simulink model "v05DCMotorHarmonicDriveTemperatureDependent"  (R2016b)
settings: Solver=VariableStepAuto  StartTime=0.0  StopTime=0.1  RelTol=1e-3  AbsTol=1e-3  EnableMultiTasking=on
values from neighbouring files (symbols this model uses):
  J_rotor = 1    [v05DCMotorHarmonicDriveTemperatureDependentScript.m]
  K_t = 0.044415    [v05DCMotorHarmonicDriveTemperatureDependentScript.m]
  V_in = 20    [v05DCMotorHarmonicDriveTemperatureDependentScript.m]
libraries: fl_lib x20, nesl_utility x10, elec_lib x1, sdl_lib x1, simulink x1
settings Model: Creator=Taeke  LastModifiedBy=Taeke
settings DataIOCC: LimitDataPoints=on
settings OptimizationCC: LifeSpan=inf
settings DebuggingCC: AllowSymbolicDim=off  SFUnexpectedBacktrackingDiag=warning  SFNoUnconditionalDefaultTransitionDiag=warning  SFExecutionAtInitializationDiag=none
settings GRTTargetCC: TargetLangStandard=C89/C90 (ANSI)  GeneratePreprocessorConditionals=Disable all
settings ConfigComp: CovMetricSettings=dw  CovHtmlReporting=on  CovSaveCumulativeToWorkspaceVar=on  CovSaveSingleToWorkspaceVar=on  CovExternalEMLEnable=off  CovSFcnEnable=off
settings SimscapeCC: SimscapeLogType=all  SimscapeLogDataHistory=10000

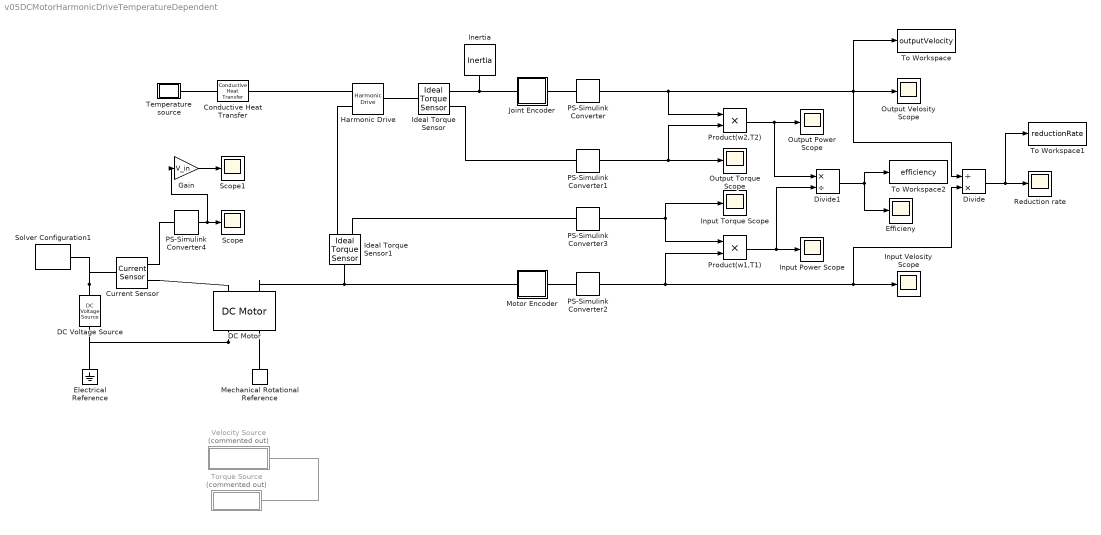
== system v05DCMotorHarmonicDriveTemperatureDependent ==
  Conductive Heat Transfer : fl_lib/Thermal/Thermal Elements/Conductive Heat Transfer  area=1 m^2  thickness=0.1 m  th_cond=401 W/(m*K)  Q_specify=off  Q_priority=None  Q=0 J/s  T_specify=off  T_priority=None  T=0 K
  Current Sensor : fl_lib/Electrical/Electrical Sensors/Current Sensor
  DC Motor : elec_lib/Actuators & Drivers/Rotational Actuators/DC Motor  parameterization=1  Ra=R_armat Ohm  La=H_armat H  emf_or_torque=2  Kv=7.2e-5 V/rpm  Ki=K_t N*m/A  T_stall=2.4e-4 N*m  w_max=1.91e+4 rpm  w_rated=1.5e+4 rpm  P_rated=0.08 W  V_rated=1.5 V  J=J_rotor g*cm^2  lam_param=1  lam=0 N*m/(rad/s)  i_noload=0 A  V_i_noload=1.5 V  speed0=0 rpm  alpha=0.00393 1/K  Tmeas=25 degC  thermal_mass=100 J/K  initial_temperature=25 degC
  DC Voltage Source : fl_lib/Electrical/Electrical Sources/DC Voltage Source  v0=V_in V
  Divide : Product  Inputs=/*
  Divide1 : Product  Inputs=*/
  Efficieny : Scope
  Electrical Reference : fl_lib/Electrical/Electrical Elements/Electrical Reference
  Gain : Gain  Gain=V_in
  Harmonic Drive : sdl_lib/Gears/Harmonic Drive  n_ellipse=N_teeth_elip  n_circle=N_teeth_circ  friction_model=1  T_noload=0.01 N*m  T_nom=0.1 N*m  efficiency_nom=.75  efficiency=0.95  mu_visc=mu N*m/(rad/s)  w_thr=0.001 rad/s  pwr_thr=P_threshold W  temperature_TLU=T_efficiency K  load_TLU=[1.0, 5.0, 10.0] N*m  efficiency_TLU=etha_efficiency  efficiency_TLU2=[0.85, 0.8, 0.75; 0.95, 0.9, 0.85; 0.85, 0.8, 0.7]  thermal_mass=C_thermal J/K  T_init=T_initial K
  Ideal Torque Sensor : fl_lib/Mechanical/Mechanical Sensors/Ideal Torque Sensor
  Ideal Torque Sensor1 : fl_lib/Mechanical/Mechanical Sensors/Ideal Torque Sensor
  Inertia : fl_lib/Mechanical/Rotational Elements/Inertia  inertia=I_load kg*m^2  w_specify=on  w_priority=High  w=0 rad/s  t_specify=off  t_priority=None  t=0 N*m
  Input Power Scope : Scope
  Input Torque Scope : Scope
  Input Velosity Scope : Scope
  Joint Encoder : Subsystem
  Mechanical Rotational Reference : fl_lib/Mechanical/Rotational Elements/Mechanical Rotational Reference
  Motor Encoder : Subsystem
  Output Power Scope : Scope
  Output Torque Scope : Scope
  Output Velosity Scope : Scope
  PS-Simulink Converter : nesl_utility/PS-Simulink Converter  PhysicalDomain=network_engine_domain  SubClassName=ps_output  LeftPortType=input  RightPortType=output  PseudoPeriodic=off  Frequencies=[]  Unit=rad/s  AffineConversion=off
  PS-Simulink Converter1 : nesl_utility/PS-Simulink Converter  PhysicalDomain=network_engine_domain  SubClassName=ps_output  LeftPortType=input  RightPortType=output  PseudoPeriodic=off  Frequencies=[]  Unit=N*m  AffineConversion=off
  PS-Simulink Converter2 : nesl_utility/PS-Simulink Converter  PhysicalDomain=network_engine_domain  SubClassName=ps_output  LeftPortType=input  RightPortType=output  PseudoPeriodic=off  Frequencies=[]  Unit=rad/s  AffineConversion=off
  PS-Simulink Converter3 : nesl_utility/PS-Simulink Converter  PhysicalDomain=network_engine_domain  SubClassName=ps_output  LeftPortType=input  RightPortType=output  PseudoPeriodic=off  Frequencies=[]  Unit=N*m  AffineConversion=off
  PS-Simulink Converter4 : nesl_utility/PS-Simulink Converter  PhysicalDomain=network_engine_domain  SubClassName=ps_output  LeftPortType=input  RightPortType=output  PseudoPeriodic=off  Frequencies=[]  Unit=A  AffineConversion=off
  Product(w1,T1) : Product
  Product(w2,T2) : Product
  Reduction rate : Scope
  Scope : Scope
  Scope1 : Scope
  Solver Configuration1 : nesl_utility/Solver Configuration  PhysicalDomain=network_engine_domain  SubClassName=solver  LeftPortType=input  RightPortType=generic  Accelerate=off  Tones=[]  Harmonics=[]  SimulateNoise=off  Profile=off  UseLocalSampling=off  EnableSwitchedLinearOptims=on  FrequencyDomain=off  UseCCode=off  RelTol=0.001  AbsTol=1e-06  MinStep=1e-09  ToWorkspace=off  RevertToSquareIcSolve=off  NumHomotopyIterations=100  PhasorMode=off  PhasorModeNumHarmonics=1  OverrideAbsTol=off  DoDC=off  ResidualTolerance=1e-09  UseLocalSolver=off  LocalSolverChoice=NE_BACKWARD_EULER_ADVANCER  LocalSolverSampleTime=0.001  DoFixedCost=off  MaxNonlinIter=3  MaxModeIter=2  LinearAlgebra=Sparse  DelaysMemoryBudget=1024  AutomaticFiltering=on  FilteringTimeConstant=0.001
  Temperature source : Subsystem  mask{Temperature=320}
      mask prompts: Temperature "Temperature [K]"
  To Workspace : ToWorkspace  VariableName=outputVelocity  SaveFormat=Timeseries  SampleTime=-1
  To Workspace1 : ToWorkspace  VariableName=reductionRate  SaveFormat=Timeseries  SampleTime=-1
  To Workspace2 : ToWorkspace  VariableName=efficiency  SaveFormat=Timeseries  SampleTime=-1
  Torque Source : Subsystem  Commented=on  mask(Rotation Velocity Source){inputTorque=2}
      mask prompts: inputTorque "Constant Torque [Nm]"
      mask help: A source which generate a constant rotational velocity.
      mask init:
      | initialVelocity = 0;
  Velocity Source : Subsystem  Commented=on  mask(Rotation Velocity Source){inputVelocity=1000}
      mask prompts: inputVelocity "Constant Velosity [rad/s]"
      mask help: A source which generate a constant rotational velocity.
      mask init:
      | initialVelocity = 0;
  wires:
  PS-Simulink Converter/1 -> Product(w2,T2)/1, Output Velosity Scope/1, To Workspace/1, Divide/1
  Divide/1 -> To Workspace1/1, Reduction rate/1
  PS-Simulink Converter2/1 -> Product(w1,T1)/2, Divide/2, Input Velosity Scope/1
  PS-Simulink Converter1/1 -> Product(w2,T2)/2, Output Torque Scope/1
  PS-Simulink Converter3/1 -> Input Torque Scope/1, Product(w1,T1)/1
  Product(w1,T1)/1 -> Divide1/2, Input Power Scope/1
  Product(w2,T2)/1 -> Divide1/1, Output Power Scope/1
  Divide1/1 -> To Workspace2/1, Efficieny/1
  PS-Simulink Converter4/1 -> Gain/1, Scope/1
  Gain/1 -> Scope1/1
  connections:
  Joint Encoder/LConn1 -- Ideal Torque Sensor/RConn1 -- Inertia/LConn1
  Joint Encoder/RConn1 -- PS-Simulink Converter/LConn1
  Motor Encoder/RConn1 -- PS-Simulink Converter2/LConn1
  Harmonic Drive/RConn1 -- Ideal Torque Sensor/LConn1
  Ideal Torque Sensor/RConn2 -- PS-Simulink Converter1/LConn1
  Ideal Torque Sensor1/RConn1 -- Harmonic Drive/LConn1
  Ideal Torque Sensor1/RConn2 -- PS-Simulink Converter3/LConn1
  Ideal Torque Sensor1/LConn1 -- DC Motor/LConn2 -- Motor Encoder/LConn1
  Conductive Heat Transfer/LConn1 -- Temperature source/RConn1
  Conductive Heat Transfer/RConn1 -- Harmonic Drive/LConn2
  DC Motor/RConn1 -- DC Voltage Source/RConn1 -- Electrical Reference/LConn1
  Mechanical Rotational Reference/LConn1 -- DC Motor/RConn2
  DC Voltage Source/LConn1 -- Solver Configuration1/RConn1 -- Current Sensor/LConn1
  Current Sensor/RConn2 -- DC Motor/LConn1
  Current Sensor/RConn1 -- PS-Simulink Converter4/LConn1
  Velocity Source/LConn1 -- Torque Source/LConn1

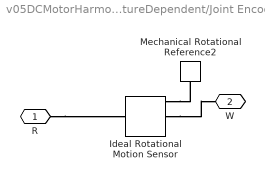
== system v05DCMotorHarmonicDriveTemperatureDependent/Joint Encoder ==
  Ideal Rotational Motion Sensor : fl_lib/Mechanical/Mechanical Sensors/Ideal Rotational Motion Sensor  offset=0 rad
  Mechanical Rotational Reference2 : fl_lib/Mechanical/Rotational Elements/Mechanical Rotational Reference
  R : PMIOPort  Port=1  Side=Left
  W : PMIOPort  Port=2  Side=Right
  connections:
  R/RConn1 -- Ideal Rotational Motion Sensor/LConn1
  Ideal Rotational Motion Sensor/RConn1 -- Mechanical Rotational Reference2/LConn1
  Ideal Rotational Motion Sensor/RConn2 -- W/RConn1

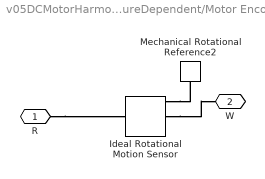
== system v05DCMotorHarmonicDriveTemperatureDependent/Motor Encoder ==
  Ideal Rotational Motion Sensor : fl_lib/Mechanical/Mechanical Sensors/Ideal Rotational Motion Sensor  offset=0 rad
  Mechanical Rotational Reference2 : fl_lib/Mechanical/Rotational Elements/Mechanical Rotational Reference
  R : PMIOPort  Port=1  Side=Left
  W : PMIOPort  Port=2  Side=Right
  connections:
  R/RConn1 -- Ideal Rotational Motion Sensor/LConn1
  Ideal Rotational Motion Sensor/RConn1 -- Mechanical Rotational Reference2/LConn1
  Ideal Rotational Motion Sensor/RConn2 -- W/RConn1

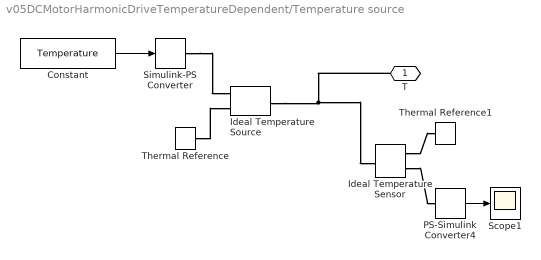
== system v05DCMotorHarmonicDriveTemperatureDependent/Temperature source ==
  Constant : Constant  Value=Temperature
  Ideal Temperature Sensor : fl_lib/Thermal/Thermal Sensors/Ideal Temperature Sensor
  Ideal Temperature Source : fl_lib/Thermal/Thermal Sources/Ideal Temperature Source
  PS-Simulink Converter4 : nesl_utility/PS-Simulink Converter  PhysicalDomain=network_engine_domain  SubClassName=ps_output  LeftPortType=input  RightPortType=output  PseudoPeriodic=off  Frequencies=[]  Unit=1  AffineConversion=off
  Scope1 : Scope
  Simulink-PS Converter : nesl_utility/Simulink-PS Converter  PhysicalDomain=network_engine_domain  SubClassName=ps_input  LeftPortType=input  RightPortType=output  PseudoPeriodic=off  Frequencies=[]  NoiseDistribution=none  NoiseParameters=[]  Unit=1  AffineConversion=off  InputFiltering=off  SimscapeFilterOrder=1  InputFilterTimeConstant=0.001  UdotUserProvided=1
  Thermal Reference : fl_lib/Thermal/Thermal Elements/Thermal Reference
  Thermal Reference1 : fl_lib/Thermal/Thermal Elements/Thermal Reference
  T : PMIOPort  Port=1  Side=Right
  wires:
  Constant/1 -> Simulink-PS Converter/1
  PS-Simulink Converter4/1 -> Scope1/1
  connections:
  Ideal Temperature Sensor/RConn1 -- Thermal Reference1/LConn1
  Simulink-PS Converter/RConn1 -- Ideal Temperature Source/RConn1
  Ideal Temperature Source/LConn1 -- T/RConn1 -- Ideal Temperature Sensor/LConn1
  Thermal Reference/LConn1 -- Ideal Temperature Source/RConn2
  Ideal Temperature Sensor/RConn2 -- PS-Simulink Converter4/LConn1

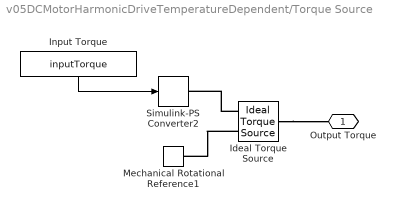
== system v05DCMotorHarmonicDriveTemperatureDependent/Torque Source ==
  Ideal Torque Source : fl_lib/Mechanical/Mechanical Sources/Ideal Torque Source
  Input Torque : Constant  Value=inputTorque
  Mechanical Rotational Reference1 : fl_lib/Mechanical/Rotational Elements/Mechanical Rotational Reference
  Simulink-PS Converter2 : nesl_utility/Simulink-PS Converter  PhysicalDomain=network_engine_domain  SubClassName=ps_input  LeftPortType=input  RightPortType=output  PseudoPeriodic=off  Frequencies=[]  NoiseDistribution=none  NoiseParameters=[]  Unit=1  AffineConversion=off  InputFiltering=off  SimscapeFilterOrder=1  InputFilterTimeConstant=0.001  UdotUserProvided=1
  Output Torque : PMIOPort  Port=1  Side=Left
  wires:
  Input Torque/1 -> Simulink-PS Converter2/1
  connections:
  Ideal Torque Source/RConn1 -- Simulink-PS Converter2/RConn1
  Ideal Torque Source/RConn2 -- Mechanical Rotational Reference1/LConn1
  Ideal Torque Source/LConn1 -- Output Torque/RConn1

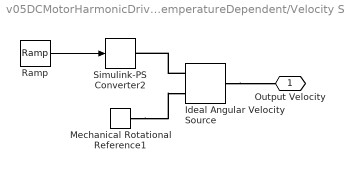
== system v05DCMotorHarmonicDriveTemperatureDependent/Velocity Source ==
  Ideal Angular Velocity Source : fl_lib/Mechanical/Mechanical Sources/Ideal Angular Velocity Source
  Mechanical Rotational Reference1 : fl_lib/Mechanical/Rotational Elements/Mechanical Rotational Reference
  Ramp : simulink/Sources/Ramp  slope=100  start=0  X0=0
  Simulink-PS Converter2 : nesl_utility/Simulink-PS Converter  PhysicalDomain=network_engine_domain  SubClassName=ps_input  LeftPortType=input  RightPortType=output  PseudoPeriodic=off  Frequencies=[]  NoiseDistribution=none  NoiseParameters=[]  Unit=1  AffineConversion=off  InputFiltering=on  SimscapeFilterOrder=1  InputFilterTimeConstant=0.001  UdotUserProvided=1
  Output Velocity : PMIOPort  Port=1  Side=Left
  wires:
  Ramp/1 -> Simulink-PS Converter2/1
  connections:
  Ideal Angular Velocity Source/RConn1 -- Simulink-PS Converter2/RConn1
  Mechanical Rotational Reference1/LConn1 -- Ideal Angular Velocity Source/RConn2
  Ideal Angular Velocity Source/LConn1 -- Output Velocity/RConn1
